simulink model "automated_tourniquet_memory_compressed2"  (R2023b)
settings: Solver=FixedStepDiscrete  StartTime=0.0  StopTime=500  FixedStep=1e-1  RelTol=1e-3  EnableMultiTasking=on
libraries: arduinolib x9, dspfdesign x3, arduinosensorlib x1
settings Model: ExtModeTrigDuration=2  Creator=doria  LastModifiedBy=doria
settings OptimizationCC: EnhancedBackFolding=on  PassReuseOutputArgsAs=Individual arguments  ZeroExternalMemoryAtStartup=off  ZeroInternalMemoryAtStartup=off  MaxStackSize=64  OptimizeBlockOrder=speed  DifferentSizesBufferReuse=on  EfficientTunableParamExpr=on
settings DebuggingCC: MultiTaskRateTransMsg=warning  ParameterTunabilityLossMsg=error
settings HardwareCC: ProdBitPerInt=16  ProdBitPerPointer=16  ProdBitPerSizeT=16  ProdBitPerPtrDiffT=16  ProdLargestAtomicFloat=None  ProdWordSize=8  ProdHWDeviceType=Atmel->AVR
settings SFSimCC: MATLABDynamicMemAlloc=off
settings RTWCC: Description=Embedded Coder  SystemTargetFile=ert.tlc  HardwareBoard=Arduino Uno  TemplateMakefile=ert_default_tmf  Toolchain=Arduino AVR  BuildConfiguration=Faster Runs
settings CodeAppCC: ForceParamTrailComments=on  IgnoreCustomStorageClasses=off  OperatorAnnotations=on  SimulinkDataObjDesc=on  SFDataObjDesc=on  InsertBlockDesc=on
settings ERTTargetCC: SupportContinuousTime=on  SupportVariableSizeSignals=on  ExtModeTransport=3  ExtModeStaticAlloc=on  ExtModeAutomaticAllocSize=off  ExtModeStaticAllocSize=250  ExtModeMexFile=ext_xcp  ExtModeIntrfLevel=Level2 - Open

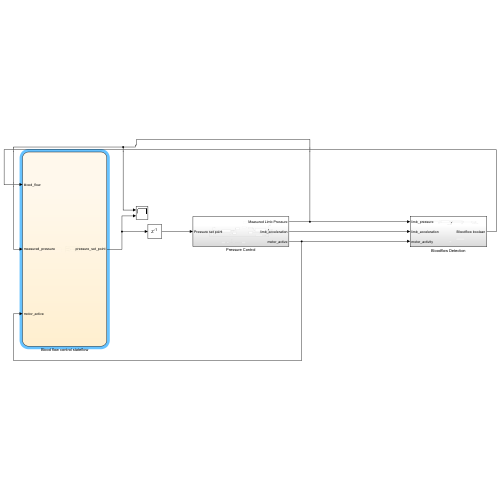
[thumbnail: Simulink's stored preview of the top-level diagram]
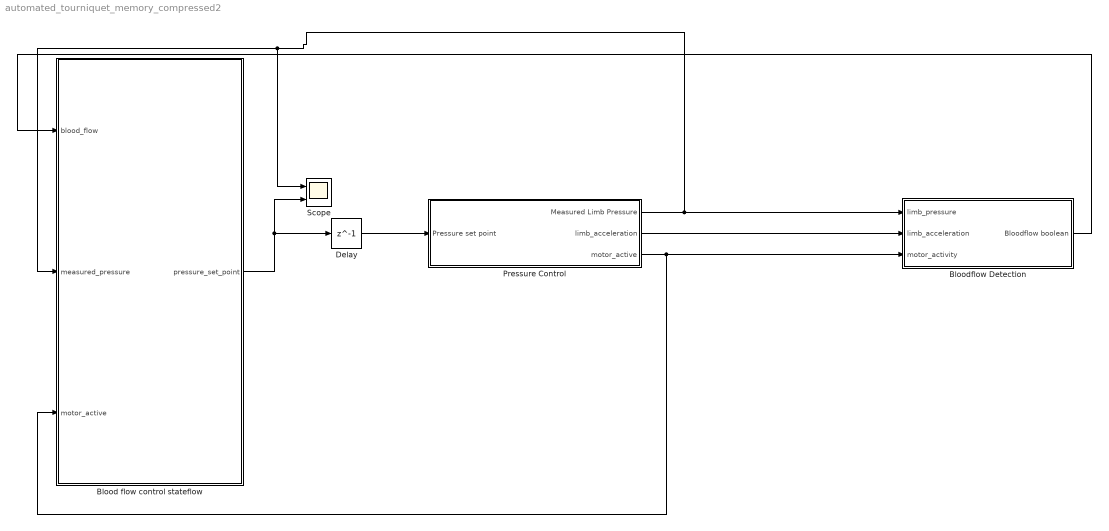
== system automated_tourniquet_memory_compressed2 ==
  Blood flow control stateflow : Stateflow chart  TreatAsAtomicUnit=on
  Bloodflow Detection : Subsystem
  Delay : Delay  DelayLength=1  InitialCondition=100
  Pressure Control : Subsystem
  Scope : Scope  NumInputPorts=2
  wires:
  Pressure Control/1(Measured Limb Pressure) -> Bloodflow Detection/1(limb_pressure), Scope/1, Blood flow control stateflow/2(measured_pressure)
  Pressure Control/3(motor_active) -> Blood flow control stateflow/3(motor_active), Bloodflow Detection/3(motor_activity)
  Bloodflow Detection/1(Bloodflow boolean) -> Blood flow control stateflow/1(blood_flow)
  Blood flow control stateflow/1(pressure_set_point) -> Delay/1, Scope/2
  Delay/1 -> Pressure Control/1(Pressure set point)
  Pressure Control/2(limb_acceleration) -> Bloodflow Detection/2(limb_acceleration)

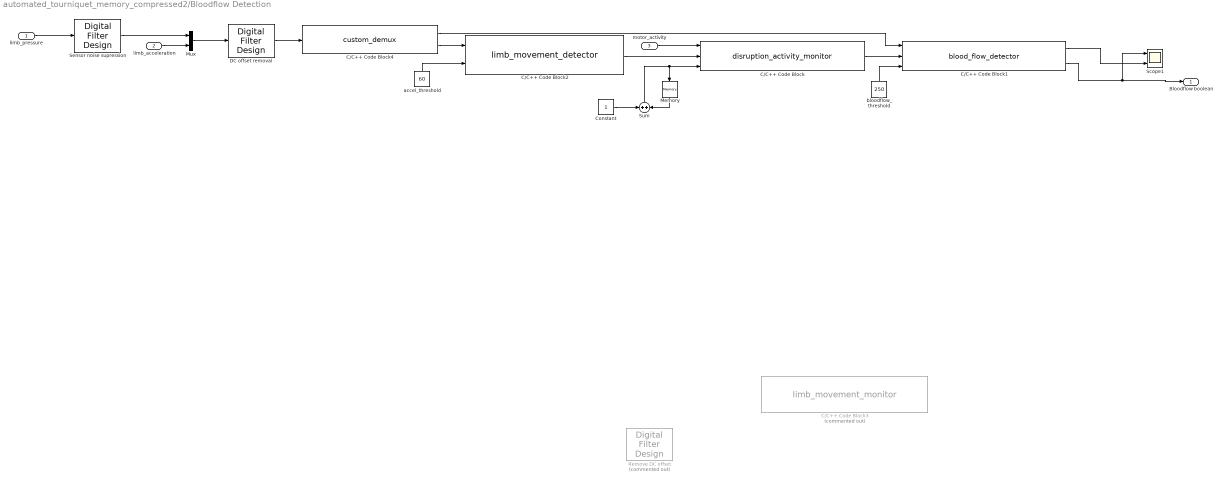
== system automated_tourniquet_memory_compressed2/Bloodflow Detection ==
  limb_pressure : Inport
  limb_acceleration : Inport  Port=2
  motor_activity : Inport  Port=3
  C/C++ Code Block : S-Function  FunctionName=disruption_activity_monitor  SFunctionModules=disruption_activity_monitor_wrapper.c  SFunctionDeploymentMode=off  EnableBusSupport=off  mask(S-Function Builder){}
      mask help: Simulink:masks:SFunctionBuilder_MD
      mask init:
      | val = [[.9  0.75 0.75 1 1 .9 .9 1]',[1 1 0.75 0.75 .9 .9 1 .9]'];try , sys = get_param(gcb,'SfunBuilderFcnName');if isempty(sys), sys = get_param(gcb,'FunctionName'); end,catch, sys = get_param(gcb,'FunctionName'); end
      settings: CopyFcn=set_param(gcbh,'LinkStatus','none')  OpenFcn=sfunctionwizard(gcbh)
      mask Display:
      | plot(val(:,1),val(:,2))
      | disp(sys)
      | port_label('input',1,'motor_active')
      | port_label('input',2,'movement_detected')
      | port_label('input',3,'time')
      | port_label('output',1,'pause_summation')
  C/C++ Code Block1 : S-Function  FunctionName=blood_flow_detector  SFunctionModules=blood_flow_detector_wrapper.c  SFunctionDeploymentMode=off  EnableBusSupport=off  mask(S-Function Builder){}
      mask help: Simulink:masks:SFunctionBuilder_MD
      mask init: same as automated_tourniquet_memory_compressed2/Bloodflow Detection/C/C++ Code Block
      settings: CopyFcn=set_param(gcbh,'LinkStatus','none')  OpenFcn=sfunctionwizard(gcbh)
      mask Display:
      | plot(val(:,1),val(:,2))
      | disp(sys)
      | port_label('input',1,'u0')
      | port_label('input',2,'disruption_active')
      | port_label('input',3,'bloodflow_threshold')
      | port_label('output',1,'y0')
      | port_label('output',2,'bloodflow_boolean')
  C/C++ Code Block2 : S-Function  FunctionName=limb_movement_detector  SFunctionModules=limb_movement_detector_wrapper.c  SFunctionDeploymentMode=off  EnableBusSupport=off  mask(S-Function Builder){}
      mask help: Simulink:masks:SFunctionBuilder_MD
      mask init: same as automated_tourniquet_memory_compressed2/Bloodflow Detection/C/C++ Code Block
      settings: CopyFcn=set_param(gcbh,'LinkStatus','none')  OpenFcn=sfunctionwizard(gcbh)
      mask Display:
      | plot(val(:,1),val(:,2))
      | disp(sys)
      | port_label('input',1,'limb_acceleration')
      | port_label('input',2,'accel_threshold')
      | port_label('output',1,'movement_boolean')
  C/C++ Code Block3 : S-Function  Commented=on  FunctionName=limb_movement_monitor  SFunctionModules=limb_movement_monitor_wrapper.c  SFunctionDeploymentMode=off  EnableBusSupport=off  mask(S-Function Builder){}
      mask help: Simulink:masks:SFunctionBuilder_MD
      mask init: same as automated_tourniquet_memory_compressed2/Bloodflow Detection/C/C++ Code Block
      settings: CopyFcn=set_param(gcbh,'LinkStatus','none')  OpenFcn=sfunctionwizard(gcbh)
      mask Display:
      | plot(val(:,1),val(:,2))
      | disp(sys)
      | port_label('input',1,'movement_detected')
      | port_label('input',2,'time')
      | port_label('output',1,'movement_cooldown')
  C/C++ Code Block4 : S-Function  FunctionName=custom_demux  SFunctionModules=custom_demux_wrapper.c  SFunctionDeploymentMode=off  EnableBusSupport=off  mask(S-Function Builder){}
      mask help: Simulink:masks:SFunctionBuilder_MD
      mask init: same as automated_tourniquet_memory_compressed2/Bloodflow Detection/C/C++ Code Block
      settings: CopyFcn=set_param(gcbh,'LinkStatus','none')  OpenFcn=sfunctionwizard(gcbh)
      mask Display:
      | plot(val(:,1),val(:,2))
      | disp(sys)
      | port_label('input',1,'combined_vector')
      | port_label('output',1,'filtered_pressure')
      | port_label('output',2,'filtered_acceleration')
  Constant : Constant  OutDataTypeStr=uint16
  DC offset removal : dspfdesign/Digital Filter Design  mwdsp_browser_bugfix_var=off
  Memory : Memory
  Mux : Mux  Inputs=2
  Remove DC offset : dspfdesign/Digital Filter Design  Commented=on  mwdsp_browser_bugfix_var=off
  Scope1 : Scope  NumInputPorts=2
  Sensor noise supression : dspfdesign/Digital Filter Design  mwdsp_browser_bugfix_var=off
  Sum : Sum  Inputs=+|+
  accel_threshold : Constant  Value=60  OutDataTypeStr=uint16
  bloodflow_threshold : Constant  Value=250  OutDataTypeStr=uint16
  Bloodflow boolean : Outport
  wires:
  Mux/1 -> DC offset removal/1
  C/C++ Code Block/1 -> C/C++ Code Block1/2
  motor_activity/1 -> C/C++ Code Block/1
  C/C++ Code Block1/2 -> Scope1/1, Bloodflow boolean/1
  bloodflow_threshold/1 -> C/C++ Code Block1/3
  C/C++ Code Block1/1 -> Scope1/2
  Constant/1 -> Sum/1
  Memory/1 -> Sum/2
  accel_threshold/1 -> C/C++ Code Block2/2
  limb_pressure/1 -> Sensor noise supression/1
  Sensor noise supression/1 -> Mux/1
  DC offset removal/1 -> C/C++ Code Block4/1
  C/C++ Code Block2/1 -> C/C++ Code Block/2
  Sum/1 -> C/C++ Code Block/3, Memory/1
  limb_acceleration/1 -> Mux/2
  C/C++ Code Block4/1 -> C/C++ Code Block1/1
  C/C++ Code Block4/2 -> C/C++ Code Block2/1

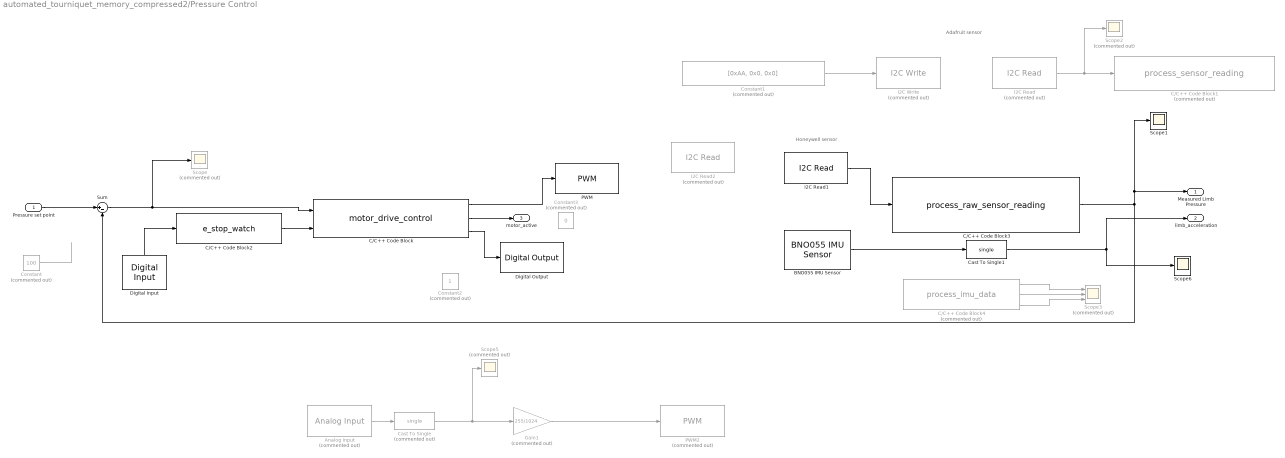
== system automated_tourniquet_memory_compressed2/Pressure Control ==
  note: Honeywell sensor
  note: Adafruit sensor
  Pressure set point : Inport
  Analog Input : arduinolib/Analog Input  Commented=on  pinNumber=0  ReadResultsOnly=off  ConversionTriggerSource=Software  ExternalTriggerType=uint32( 0 )  OutputDataType=uint16  EnableConversionCompleteNotify=off  EnableOuputStatus=off  SampleTime=-1  blockPlatform=arduino
  BNO055 IMU Sensor : arduinosensorlib/BNO055 IMU Sensor  SlaveAddress=0x29  OperationMode=Fusion  Accel=on  AngularRate=off  MagField=off  EulerAngles=off  Quat=off  LinearAccel=off  GravityVector=off  Status=off  Timestamp=off  AccelRange=4G  AccelBW=62.5 Hz  GyroRange=2000 dps  GyroBW=32 Hz  MagODR=10 Hz  spf=1  SampleTime=-1  blockPlatform=ARDUINO  QueueSizeFactor=1
  C/C++ Code Block : S-Function  FunctionName=motor_drive_control  SFunctionModules=motor_drive_control_wrapper.c  SFunctionDeploymentMode=off  EnableBusSupport=off  mask(S-Function Builder){}
      mask help: Simulink:masks:SFunctionBuilder_MD
      mask init: same as automated_tourniquet_memory_compressed2/Bloodflow Detection/C/C++ Code Block
      settings: CopyFcn=set_param(gcbh,'LinkStatus','none')  OpenFcn=sfunctionwizard(gcbh)
      mask Display:
      | plot(val(:,1),val(:,2))
      | disp(sys)
      | port_label('input',1,'limb_pressure_diff')
      | port_label('input',2,'emergency_stop')
      | port_label('output',1,'inflation_state')
      | port_label('output',2,'motor_active')
      | port_label('output',3,'solenoid_state')
  C/C++ Code Block1 : S-Function  Commented=on  FunctionName=process_sensor_reading  SFunctionModules=process_sensor_reading_wrapper.c  SFunctionDeploymentMode=off  EnableBusSupport=off  mask(S-Function Builder){}
      mask help: Simulink:masks:SFunctionBuilder_MD
      mask init: same as automated_tourniquet_memory_compressed2/Bloodflow Detection/C/C++ Code Block
      settings: CopyFcn=set_param(gcbh,'LinkStatus','none')  OpenFcn=sfunctionwizard(gcbh)
      mask Display:
      | plot(val(:,1),val(:,2))
      | disp(sys)
      | port_label('input',1,'sensor_reading')
      | port_label('output',1,'processed_output')
  C/C++ Code Block2 : S-Function  FunctionName=e_stop_watch  SFunctionModules=e_stop_watch_wrapper.c  SFunctionDeploymentMode=off  EnableBusSupport=off  mask(S-Function Builder){}
      mask help: Simulink:masks:SFunctionBuilder_MD
      mask init: same as automated_tourniquet_memory_compressed2/Bloodflow Detection/C/C++ Code Block
      settings: CopyFcn=set_param(gcbh,'LinkStatus','none')  OpenFcn=sfunctionwizard(gcbh)
      mask Display:
      | plot(val(:,1),val(:,2))
      | disp(sys)
      | port_label('input',1,'arduino_input')
      | port_label('output',1,'estop')
  C/C++ Code Block3 : S-Function  FunctionName=process_raw_sensor_reading  SFunctionModules=process_raw_sensor_reading_wrapper.c  SFunctionDeploymentMode=off  EnableBusSupport=off  mask(S-Function Builder){}
      mask help: Simulink:masks:SFunctionBuilder_MD
      mask init: same as automated_tourniquet_memory_compressed2/Bloodflow Detection/C/C++ Code Block
      settings: CopyFcn=set_param(gcbh,'LinkStatus','none')  OpenFcn=sfunctionwizard(gcbh)
      mask Display:
      | plot(val(:,1),val(:,2))
      | disp(sys)
      | port_label('input',1,'raw_sensor_input')
      | port_label('output',1,'limb_pressure_mmhg')
  C/C++ Code Block4 : S-Function  Commented=on  FunctionName=process_imu_data  SFunctionModules=process_imu_data_wrapper.c  SFunctionDeploymentMode=off  EnableBusSupport=off  mask(S-Function Builder){}
      mask help: Simulink:masks:SFunctionBuilder_MD
      mask init: same as automated_tourniquet_memory_compressed2/Bloodflow Detection/C/C++ Code Block
      settings: CopyFcn=set_param(gcbh,'LinkStatus','none')  OpenFcn=sfunctionwizard(gcbh)
      mask Display:
      | plot(val(:,1),val(:,2))
      | disp(sys)
      | port_label('input',1,'raw_imu_input')
      | port_label('output',1,'x_angle')
      | port_label('output',2,'y_angle')
      | port_label('output',3,'z_angle')
  Cast To Single : DataTypeConversion  Commented=on  OutDataTypeStr=single  SaturateOnIntegerOverflow=off  RndMeth=Floor
  Cast To Single1 : DataTypeConversion  OutDataTypeStr=single  SaturateOnIntegerOverflow=off  RndMeth=Floor
  Constant : Constant  Commented=on  Value=100  OutDataTypeStr=single
  Constant1 : Constant  Commented=on  Value=[0xAA, 0x0, 0x0]  OutDataTypeStr=uint8
  Constant2 : Constant  Commented=on  OutDataTypeStr=boolean
  Constant3 : Constant  Commented=on  Value=0  OutDataTypeStr=boolean
  Digital Input : arduinolib/Digital Input  pinNumber=4  mode=Default  Direction=input  SampleTime=0.1  blockPlatform=arduino
  Digital Output : arduinolib/Digital Output  pinNumber=2  Direction=output  blockPlatform=arduino
  Gain1 : Gain  Commented=on  Gain=255/1024  ParamDataTypeStr=single
  I2C Read : arduinolib/I2C Read  Commented=on  I2CModule=0  Mode=Master  SlaveAddress=0x18  SlaveByteOrder=BigEndian  Direction=Receiver  RegisterAddressMode=off  RegisterAddress=0  SlaveDataType=uint8  DataLength=4  NoAck=off  RepeatedStart=off  OutputStatus=off  blockPlatform=ARDUINO  SampleTime=0.1
  I2C Read1 : arduinolib/I2C Read  I2CModule=0  Mode=Master  SlaveAddress=0x28  SlaveByteOrder=BigEndian  Direction=Receiver  RegisterAddressMode=off  RegisterAddress=1  SlaveDataType=uint8  DataLength=2  NoAck=off  RepeatedStart=off  OutputStatus=off  blockPlatform=ARDUINO  SampleTime=0.1
  I2C Read2 : arduinolib/I2C Read  Commented=on  I2CModule=0  Mode=Master  SlaveAddress=0x29  SlaveByteOrder=BigEndian  Direction=Receiver  RegisterAddressMode=on  RegisterAddress=8  SlaveDataType=uint8  DataLength=6  NoAck=off  RepeatedStart=off  OutputStatus=off  blockPlatform=ARDUINO  SampleTime=0.1
  I2C Write : arduinolib/I2C Write  Commented=on  I2CModule=0  Mode=Master  SlaveAddress=0x18  SlaveByteOrder=BigEndian  Direction=Transmitter  RegisterAddressMode=off  RegisterAddress=0  SlaveDataType=uint8  DataLength=1  NoAck=off  RepeatedStart=on  OutputStatus=off  blockPlatform=ARDUINO
  PWM : arduinolib/PWM  pinNumber=3  frequencyType=Default  desiredFrequency=490.2  achievableFrequency=490.2
  PWM2 : arduinolib/PWM  Commented=on  pinNumber=3  frequencyType=Default  desiredFrequency=490.2  achievableFrequency=490.2
  Scope : Scope  Commented=on
  Scope1 : Scope
  Scope2 : Scope  Commented=on
  Scope3 : Scope  Commented=on  NumInputPorts=3
  Scope5 : Scope  Commented=on
  Scope6 : Scope
  Sum : Sum  Inputs=|+-
  Measured Limb Pressure : Outport
  limb_acceleration : Outport  Port=2
  motor_active : Outport  Port=3
  wires:
  I2C Read/1 -> Scope2/1, C/C++ Code Block1/1
  Constant1/1 -> I2C Write/1
  Analog Input/1 -> Cast To Single/1
  Gain1/1 -> PWM2/1
  C/C++ Code Block3/1 -> Sum/2, Scope1/1, Measured Limb Pressure/1
  C/C++ Code Block/1 -> PWM/1
  Cast To Single/1 -> Scope5/1, Gain1/1
  Digital Input/1 -> C/C++ Code Block2/1
  C/C++ Code Block2/1 -> C/C++ Code Block/2
  C/C++ Code Block/2 -> motor_active/1
  C/C++ Code Block/3 -> Digital Output/1
  Constant/1 -> ?
  I2C Read1/1 -> C/C++ Code Block3/1
  C/C++ Code Block4/2 -> Scope3/2
  C/C++ Code Block4/1 -> Scope3/1
  C/C++ Code Block4/3 -> Scope3/3
  BNO055 IMU Sensor/1 -> Cast To Single1/1
  Cast To Single1/1 -> Scope6/1, limb_acceleration/1
  Pressure set point/1 -> Sum/1
  Sum/1 -> Scope/1, C/C++ Code Block/1

== stateflow chart automated_tourniquet_memory_compressed2/Blood flow control stateflow ==
  settings: updateMethod=DISCRETE  sampleTime=0.1
  state Binary_search_ideal_pressure
    % Find ideal pressure to stop bleeding between pressure extremes measured in previous stage
    entry:
    binary_search_upper = 250 %pressure_upper_bound
    binary_search_lower = 100 %pressure_lower_bound
    ideal_pressure_found = false
    state Too_tight
      entry:
      binary_search_upper = pressure_set_point
    state Adjust_pressure_set_point
      entry:
      pressure_set_point = (binary_search_upper + binary_search_lower)/2
      pressure_difference = binary_search_upper - binary_search_lower
    state Ideal_pressure_found
      entry:
      pressure_set_point = binary_search_upper
      ideal_pressure_found = true
    state Idle
    state Too_loose
      entry:
      binary_search_lower = pressure_set_point
    Too_tight -> Adjust_pressure_set_point
    (junction 112) -> Too_tight [order 3] : [pressure_difference >= 30 ...
        |  && blood_flow == 0]
    (default) -> Adjust_pressure_set_point
    (junction 112) -> Ideal_pressure_found [order 1] : [pressure_difference < 30]
    Binary_search_ideal_pressure.Idle -> (junction 112) : [duration(motor_active == 0) > 5]
    Adjust_pressure_set_point -> Binary_search_ideal_pressure.Idle : [(measured_pressure >= pressure_set_point - 30/2) ...
        | && (measured_pressure  <= pressure_set_point + 30/2)]
    (junction 112) -> Too_loose [order 2] : [pressure_difference >= 30 ...
        |  && blood_flow > 0]
    Too_loose -> Adjust_pressure_set_point
  state Find_initial_bounds [commented out]
    entry:
    pressure_set_point = 100
    upper_bound_found = false
    state Inflate [commented out]
      %Inflate quickly to stop blood flow
      exit:
      pressure_upper_bound = pressure_set_point
      state Initial_wait [commented out]
        % Used to wait out the
        % initial to ensure all
        % data signals are acccurate
        %entry:
        %initial_inflation = true
        %exit:
        %initial_inflation = false
      state Idle [commented out]
      state Increase_pressure_set_point [commented out]
        entry:
        pressure_set_point = pressure_set_point + 30 %bulk_increment
      state wait [commented out]
      (default) -> Initial_wait [commented out]
      Find_initial_bounds.Inflate.Idle -> Increase_pressure_set_point [commented out] : [duration(motor_active == 0) > 10]
      wait -> Find_initial_bounds.Inflate.Idle [commented out] : [measured_pressure >= pressure_set_point]
      Increase_pressure_set_point -> wait [commented out]
      Initial_wait -> wait [commented out] : after(1.5,sec)
    state Deflate [commented out]
      % Slowly deflate until blood flow returns
      exit:
      pressure_lower_bound = pressure_set_point
      state Idle [commented out]
      state Decrease_pressure_set_point [commented out]
        entry:
        pressure_set_point = pressure_set_point - 30 %bulk_decrement
      state Wait [commented out]
      (default) -> Decrease_pressure_set_point [commented out]
      Wait -> Find_initial_bounds.Deflate.Idle [commented out] : [measured_pressure<=pressure_set_point]
      Find_initial_bounds.Deflate.Idle -> Decrease_pressure_set_point [commented out] : [duration(motor_active == 0) > 10]
      Decrease_pressure_set_point -> Wait [commented out]
    note: 1.5 seconds is for the transport delay
    (default) -> Inflate [commented out]
    Inflate -> Deflate [commented out] : [duration(blood_flow == 0) > 5]{upper_bound_found = true}
  state Fine_adjustments [commented out]
    state Increase_pressure [commented out]
      entry:
      pressure_set_point = pressure_set_point + 10 %fine_increment
    state idle [commented out]
    state Default_state [commented out]
    state Decrease_pressure [commented out]
      entry:
      pressure_set_point = pressure_set_point - 10 %fine_decrement
    Default_state -> Increase_pressure [commented out] : [duration(blood_flow>0) > 5]
    (default) -> Default_state [commented out]
    Increase_pressure -> idle [commented out]
    idle -> Default_state [commented out] : [duration(motor_active == 0) > 10]
    Decrease_pressure -> idle [commented out]
    Default_state -> Decrease_pressure [commented out] : [duration(blood_flow ==0) > 5]
  state Idle [commented out]
    % Wait in the idle state for a given amount of time
  (default) -> Binary_search_ideal_pressure
  (default) -> Find_initial_bounds [commented out]
  Fine_adjustments -> Idle [commented out] : [duration(blood_flow == 0) > 10 && [duration(motor_active == 0) > 10]]
  Binary_search_ideal_pressure -> Idle [commented out] : [ideal_pressure_found==true]
  Find_initial_bounds -> Binary_search_ideal_pressure [commented out] : [(duration(blood_flow>0) > 4) && upper_bound_found == true]
  Idle -> Fine_adjustments [commented out] : [duration(blood_flow > 0) > 10]
  data: pressure_set_point output single; blood_flow input; measured_pressure input single; binary_search_lower local single; binary_search_upper local single; ideal_pressure_found local boolean; pressure_difference local single; pressure_lower_bound local single; pressure_upper_bound local single; upper_bound_found local boolean; motor_active input boolean
